simulink model "simulink_in_stateflow"  (R2015b)
settings: Solver=VariableStepAuto  StartTime=0.0  StopTime=10.0  RelTol=1e-3
settings Model: Creator=ladmin  LastModifiedBy=ladmin

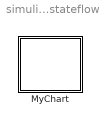
== system simulink_in_stateflow ==
  MyChart : Stateflow chart  TreatAsAtomicUnit=on

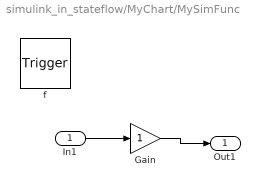
== system simulink_in_stateflow/MyChart/MySimFunc ==
  In1 : Inport
  f : TriggerPort  TriggerType=function-call
      settings: CopyFcn=Stateflow.SLINSF.SimulinkMan.removeBlockPreDeleteFcn  PreDeleteFcn=Stateflow.SLINSF.SimulinkMan.unsafePredeleteFcn
  Gain : Gain
  Out1 : Outport
  wires:
  In1/1 -> Gain/1
  Gain/1 -> Out1/1

== stateflow chart simulink_in_stateflow/MyChart ==
  state MyState1
  state MyState2
  state Out1 = MySimFunc(In1) [function]
  MyState1 -> (junction 4)
  data: In1 function_input; Out1 function_output
